simulink model "Lab4"  (R2024a)
settings: Solver=VariableStepAuto  StartTime=0.0  StopTime=100  RelTol=1e-3
settings Model: Creator=Pawel  LastModifiedBy=Pawel

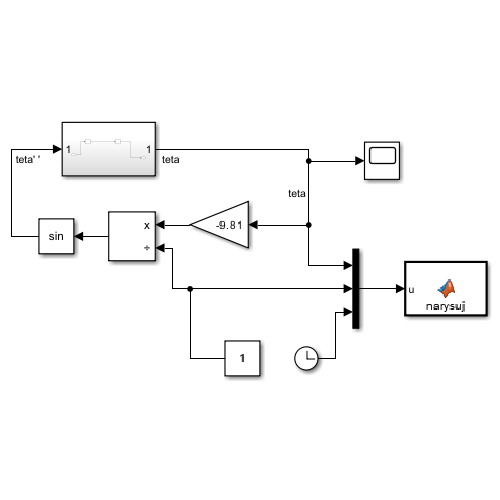
[thumbnail: Simulink's stored preview of the top-level diagram]
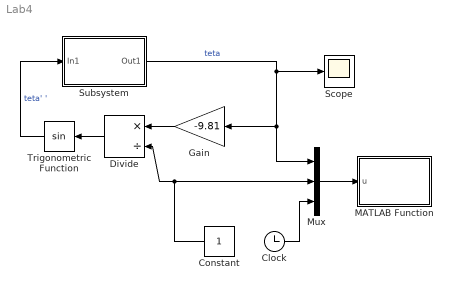
== system Lab4 ==
  Clock : Clock
  Constant : Constant
  Divide : Product  Inputs=*/
  Gain : Gain  Gain=-9.81
  MATLAB Function : MATLAB Function  TreatAsAtomicUnit=on
  Mux : Mux  Inputs=3
  Scope : Scope
  Subsystem : Subsystem
  Trigonometric Function : Trigonometry
  wires:
  Subsystem/1(Out1) -> Scope/1, Mux/1, Gain/1  "teta"
  Constant/1 -> Mux/2, Divide/2
  Clock/1 -> Mux/3
  Mux/1 -> MATLAB Function/1(u)
  Gain/1 -> Divide/1
  Divide/1 -> Trigonometric Function/1
  Trigonometric Function/1 -> Subsystem/1(In1)  "teta' '"

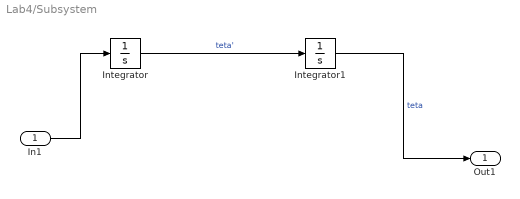
== system Lab4/Subsystem ==
  In1 : Inport
  Integrator : Integrator
  Integrator1 : Integrator  InitialCondition=0.1
  Out1 : Outport
  wires:
  Integrator/1 -> Integrator1/1  "teta'"
  In1/1 -> Integrator/1
  Integrator1/1 -> Out1/1  "teta"

== matlab function Lab4/MATLAB Function ==
  data: u input
function narysuj(u)

teta = u(1);
l = u(2);
t = u(3);

y=-l*cos(teta);
x=l*sin(teta);

cla
fill([-1/4 -1/4 1/4 1/4],[0.1 0 0 0.1],'r')
hold on;
line([0 x],[0 y])
plot(x,y,'r.','MarkerSize',30)
xlim([-l l])
ylim([-l 0.1])
text(-1/4,0.005,["  T = "])
hold off
axis off

drawnow
